simulink model "nonmininumS"  (R2018b)
settings: Solver=VariableStepAuto  StartTime=0.0  StopTime=Tsim  MaxStep=0.01  RelTol=1e-3
values from neighbouring files (symbols this model uses):
  A = A'    [ex2_fu.m]    (also in fu.m = fliplr(flipud(A)))
  B = B'    [ex2_fu.m]    (also in fu.m = flipud(B)*b0)
  C = C'    [ex2_fu.m]    (also in fu.m = fliplr(C)/b0)
  d = round(L/Ts)    [ex2_fu.m]
  kr = inv([1 0]*inv(eye(2)-A+B*K)*B)    [ex2_fu.m]
  Tpert = 10    [ex2_fu.m]
  Truido = 20    [ex2_fu.m]
  Ts = 0.05    [ex2_fu.m]
libraries: cstblocks x5, simulink x1
settings Model: Creator=Bismark  LastModifiedBy=rene
settings DebuggingCC: LibraryContextMissingDiagnostic=none
settings SFSimCC: SimUseLocalCustomCode=off
settings RTWCC: RTWUseLocalCustomCode=off
settings CodeAppCC: StateflowObjectComments=on

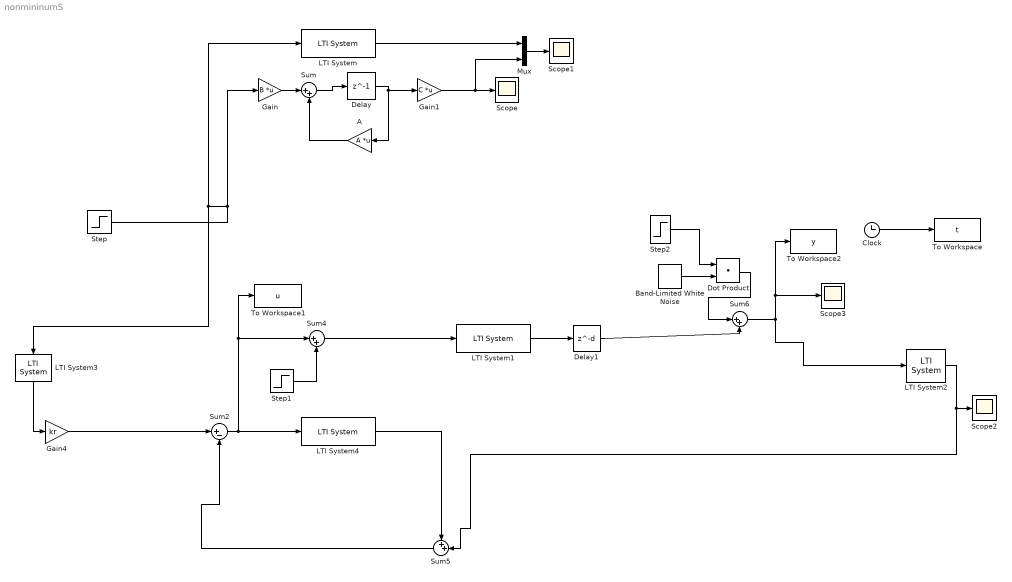
== system nonmininumS ==
  A : Gain  Gain=A  Multiplication=Matrix(K*u) (u vector)
  Band-Limited White Noise : simulink/Sources/Band-Limited White Noise  Cov=1e-7  Ts=Ts  seed=[23341]
  Clock : Clock
  Delay : Delay  DelayLength=1  SampleTime=Ts
  Delay1 : Delay  DelayLength=d  SampleTime=Ts
  Dot Product : DotProduct  InputSameDT=on  OutDataTypeStr=Inherit: Inherit via internal rule
  Gain : Gain  Gain=B  Multiplication=Matrix(K*u) (u vector)
  Gain1 : Gain  Gain=C  Multiplication=Matrix(K*u)
  Gain4 : Gain  Gain=kr
  LTI System : cstblocks/LTI System  sys=G  IC=[]
  LTI System1 : cstblocks/LTI System  sys=Gpd  IC=[]
  LTI System2 : cstblocks/LTI System  sys=V  IC=[]
  LTI System3 : cstblocks/LTI System  sys=Fr  IC=[]
  LTI System4 : cstblocks/LTI System  sys=S  IC=[]
  Mux : Mux  Inputs=2
  Scope{,1..3} (4 alike) : Scope
  Step : Step  Time=0  SampleTime=0
  Step1 : Step  Time=Tpert  After=-1  SampleTime=Ts
  Step2 : Step  Time=Truido  SampleTime=0
  Sum : Sum  Inputs=|++
  Sum2 : Sum  Inputs=|+-
  Sum4 : Sum  Inputs=|++
  Sum5 : Sum  Inputs=++|
  Sum6 : Sum  Inputs=|++
  To Workspace : ToWorkspace  VariableName=t  SampleTime=Ts
  To Workspace1 : ToWorkspace  VariableName=u  SampleTime=Ts
  To Workspace2 : ToWorkspace  VariableName=y  SampleTime=Ts
  wires:
  Step/1 -> LTI System/1, LTI System3/1, Gain/1
  Gain/1 -> Sum/1
  A/1 -> Sum/2
  Sum/1 -> Delay/1
  Delay/1 -> A/1, Gain1/1
  Gain1/1 -> Mux/2, Scope/1
  LTI System/1 -> Mux/1
  Mux/1 -> Scope1/1
  Sum2/1 -> LTI System4/1, Sum4/1, To Workspace1/1
  Gain4/1 -> Sum2/1
  Clock/1 -> To Workspace/1
  Step1/1 -> Sum4/2
  Sum5/1 -> Sum2/2
  Sum6/1 -> LTI System2/1, Scope3/1, To Workspace2/1
  LTI System2/1 -> Sum5/2, Scope2/1
  LTI System3/1 -> Gain4/1
  Step2/1 -> Dot Product/1
  Band-Limited White Noise/1 -> Dot Product/2
  Dot Product/1 -> Sum6/1
  LTI System4/1 -> Sum5/1
  LTI System1/1 -> Delay1/1
  Delay1/1 -> Sum6/2
  Sum4/1 -> LTI System1/1
